simulink model "Ev3Model"  (R2019a)
settings: Solver=VariableStepAuto  StartTime=0.0  StopTime=40  RelTol=1e-3
values from neighbouring files (symbols this model uses):
  A = [0 1 0 0 ... (first row only)    [BEST.m]    (also in EV3Plant.m)
  Ac = A-B*K    [BEST.m]    (also in EV3Plant.m)
  B = [0;-m*l/d;0;(I+m*l^2)/d]    [BEST.m]    (also in EV3Plant.m)
  C = [1 0 0 0 ... (first row only)    [BEST.m]    (also in EV3Plant.m)
  D = [0 ... (first row only)    [BEST.m]    (also in EV3Plant.m)
  K = -[23.0811,2.5151,0.3162,1.0021]    [BEST.m]    (also in EV3Plant.m = lqr(A,B,Q,R))
  Kd = 0.005    [BEST.m]    (also in EV3Plant.m)
  Ki = 0.5    [BEST.m]    (also in EV3Plant.m)
  Kp = 1.5    [BEST.m]    (also in EV3Plant.m)
libraries: simulink x3
settings Model: Creator=mikiz  LastModifiedBy=mikiz
settings SolverCC: MaxConsecutiveMinStep=3  AlgebraicLoopSolver=LineSearch
settings DataIOCC: ReturnWorkspaceOutputs=off
settings DebuggingCC: ArithmeticOperatorsInVariantConditions=warning

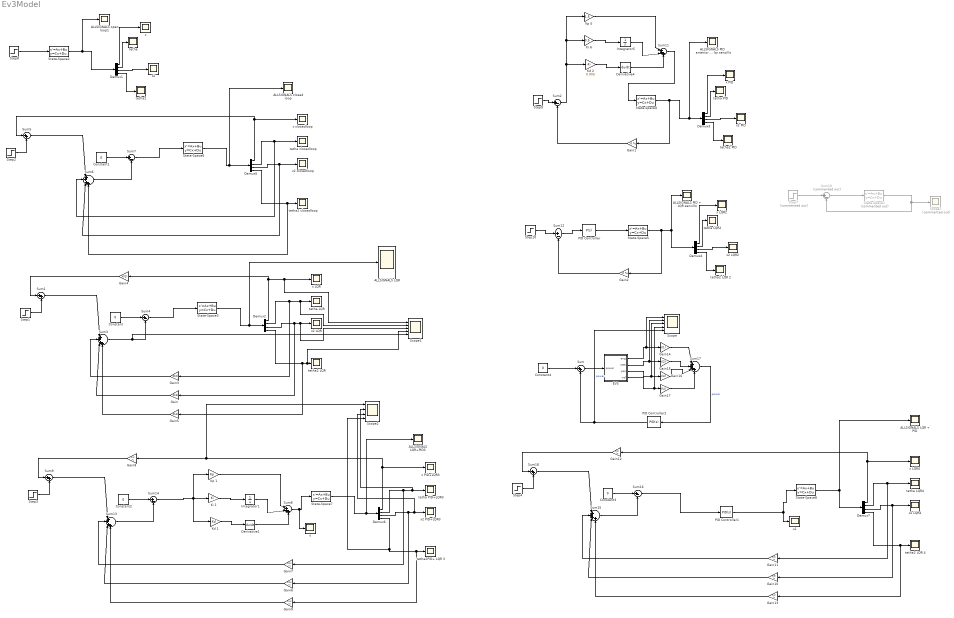
== system Ev3Model ==
  ALLSIGNALS LQR + PID : Scope
  "ALLSIGNALS PID + LQR sencillo " : Scope
  ALLSIGNALS PID anterior + lqr sencillo : Scope
  "ALLSIGNALS LQR " : Scope
  "ALLSIGNALS LQR+PIDS " : Scope
  ALLSIGNALS closed loop : Scope
  ALLSIGNALS open loop1 : Scope
  Constant{,1..4} (5 alike) : Constant  Value=0
  Demux{1..7} (7 alike) : Demux
  Derivative1 : Derivative
  Derivative4 : Derivative
  "EV3 " : Subsystem
  Gain : Gain  Gain=K(3)
  Gain1 : Gain  Gain=K  Multiplication=Matrix(K*u)
  Gain10 : Gain  Gain=K(3)  Multiplication=Matrix(K*u)
  Gain11 : Gain  Gain=K(2)  Multiplication=Matrix(K*u)
  Gain12 : Gain  Gain=K(1)  Multiplication=Matrix(K*u)
  Gain13 : Gain  Gain=K(4)  Multiplication=Matrix(K*u)
  Gain14 : Gain  Gain=K(1)
  Gain15 : Gain  Gain=K(2)
  Gain16 : Gain  Gain=K(3)
  Gain17 : Gain  Gain=K(4)
  Gain2 : Gain  Gain=K  Multiplication=Matrix(K*u)
  Gain3 : Gain  Gain=K(2)
  Gain4 : Gain  Gain=K(1)
  Gain5 : Gain  Gain=K(4)
  Gain6 : Gain  Gain=K(3)  Multiplication=Matrix(K*u)
  Gain7 : Gain  Gain=K(2)  Multiplication=Matrix(K*u)
  Gain8 : Gain  Gain=K(1)  Multiplication=Matrix(K*u)
  Gain9 : Gain  Gain=K(4)  Multiplication=Matrix(K*u)
  Integrator1 : Integrator
  Integrator5 : Integrator
  Kd 1 : Gain  Gain=Kd
  Kd 2 : Gain  Gain=0.005
  Ki 1 : Gain  Gain=Ki
  Ki 6 : Gain  Gain=0.5
  Kp 1 : Gain  Gain=Kp
  Kp 5 : Gain  Gain=1.5
  PID Controller : simulink/Continuous/PID Controller  Controller=P  Form=Parallel  TimeDomain=Continuous-time  SampleTime=-1  IntegratorMethod=Forward Euler  FilterMethod=Forward Euler  ControllerParametersSource=internal  P=25  I=0  D=0  UseFilter=on  N=100  TunerSelectOption=Transfer Function Based (PID Tuner App)  InitialConditionSource=internal  InitialConditionForIntegrator=0  InitialConditionForFilter=0  DifferentiatorICPrevScaledInput=0  ExternalReset=none  TrackingMode=off  Kt=1  LimitOutput=off  UpperSaturationLimit=inf  LowerSaturationLimit=-inf  LinearizeAsGain=on  AntiWindupMode=none  Kb=1  POutMin=[]  POutMax=[]  IOutMin=[]  IOutMax=[]  DOutMin=[]  DOutMax=[]  NOutMin=[]  NOutMax=[]  SumOutMin=[]  SumOutMax=[]  SaturationOutMin=[]  SaturationOutMax=[]  PParamMin=[]  PParamMax=[]  IParamMin=[]  IParamMax=[]  DParamMin=[]  DParamMax=[]  NParamMin=[]  NParamMax=[]  KbParamMin=[]  KbParamMax=[]  KtParamMin=[]  KtParamMax=[]  KbOutMin=[]  KbOutMax=[]  KtOutMin=[]  KtOutMax=[]  IntegratorOutMin=[]  IntegratorOutMax=[]  FilterOutMin=[]  FilterOutMax=[]  SumI1OutMin=[]  SumI1OutMax=[]  SumI2OutMin=[]  SumI2OutMax=[]  SumI3OutMin=[]  SumI3OutMax=[]  SumI4OutMin=[]  SumI4OutMax=[]  SumDOutMin=[]  SumDOutMax=[]  DifferentiatorOutMin=[]  DifferentiatorOutMax=[]  FilterDiffOutCoefMin=[]  FilterDiffOutCoefMax=[]  ReciprocalOutMin=[]  ReciprocalOutMax=[]  SumDenOutMin=[]  SumDenOutMax=[]  SumNumOutMin=[]  SumNumOutMax=[]  DivideOutMin=[]  DivideOutMax=[]  IntegratorContinuousStateAttributes=''  IntegratorStateMustResolveToSignalObject=off  IntegratorRTWStateStorageClass=Auto  FilterContinuousStateAttributes=''  FilterStateMustResolveToSignalObject=off  FilterRTWStateStorageClass=Auto  ParallelPVariant=InternalParameters  IdealPVariant=Disabled  IVariant=Disabled  DVariant=Disabled  IntegratorVariant=Disabled  SatVariant=Disabled  AWVariant=Disabled  PCopyVariant=Disabled  TRVariant=Disabled  FdbkBlocksVariant=Forward  IdealPFdbkVariant=Disabled  SatFdbkVariant=Disabled  DerivativeFilterVariant=Disabled  NVariant=Disabled  NCopyVariant=Disabled_SignalSpec  FilterICVariant=Disabled  IntegratorICVariant=Disabled  ExternalResetVariant=Disabled  TRSumVariant=Passthrough  SumFdbkVariant=Disabled  SumVariant=Passthrough_P
  PID Controller1 : simulink/Continuous/PID Controller  Controller=PID  Form=Parallel  TimeDomain=Continuous-time  SampleTime=-1  IntegratorMethod=Forward Euler  FilterMethod=Forward Euler  ControllerParametersSource=internal  P=3.727  I=24.1  D=-0.01253  UseFilter=on  N=66.27  TunerSelectOption=Transfer Function Based (PID Tuner App)  InitialConditionSource=internal  InitialConditionForIntegrator=0  InitialConditionForFilter=0  DifferentiatorICPrevScaledInput=0  ExternalReset=none  TrackingMode=off  Kt=1  LimitOutput=off  UpperSaturationLimit=inf  LowerSaturationLimit=-inf  LinearizeAsGain=on  AntiWindupMode=none  Kb=1  POutMin=[]  POutMax=[]  IOutMin=[]  IOutMax=[]  DOutMin=[]  DOutMax=[]  NOutMin=[]  NOutMax=[]  SumOutMin=[]  SumOutMax=[]  SaturationOutMin=[]  SaturationOutMax=[]  PParamMin=[]  PParamMax=[]  IParamMin=[]  IParamMax=[]  DParamMin=[]  DParamMax=[]  NParamMin=[]  NParamMax=[]  KbParamMin=[]  KbParamMax=[]  KtParamMin=[]  KtParamMax=[]  KbOutMin=[]  KbOutMax=[]  KtOutMin=[]  KtOutMax=[]  IntegratorOutMin=[]  IntegratorOutMax=[]  FilterOutMin=[]  FilterOutMax=[]  SumI1OutMin=[]  SumI1OutMax=[]  SumI2OutMin=[]  SumI2OutMax=[]  SumI3OutMin=[]  SumI3OutMax=[]  SumI4OutMin=[]  SumI4OutMax=[]  SumDOutMin=[]  SumDOutMax=[]  DifferentiatorOutMin=[]  DifferentiatorOutMax=[]  FilterDiffOutCoefMin=[]  FilterDiffOutCoefMax=[]  ReciprocalOutMin=[]  ReciprocalOutMax=[]  SumDenOutMin=[]  SumDenOutMax=[]  SumNumOutMin=[]  SumNumOutMax=[]  DivideOutMin=[]  DivideOutMax=[]  IntegratorContinuousStateAttributes=''  IntegratorStateMustResolveToSignalObject=off  IntegratorRTWStateStorageClass=Auto  FilterContinuousStateAttributes=''  FilterStateMustResolveToSignalObject=off  FilterRTWStateStorageClass=Auto  ParallelPVariant=InternalParameters  IdealPVariant=Disabled  IVariant=InternalParameters  DVariant=InternalParameters  IntegratorVariant=Continuous  SatVariant=Disabled  AWVariant=Passthrough  PCopyVariant=Disabled  TRVariant=Disabled  FdbkBlocksVariant=Forward  IdealPFdbkVariant=Disabled  SatFdbkVariant=Disabled  DerivativeFilterVariant=ContFilter  NVariant=InternalParameters  NCopyVariant=Disabled  FilterICVariant=InternalICsFilter  IntegratorICVariant=InternalICs  ExternalResetVariant=Disabled  TRSumVariant=Passthrough  SumFdbkVariant=Disabled  SumVariant=Sum_PID
  PID Controller2 : simulink/Continuous/PID Controller  Controller=PID  Form=Parallel  TimeDomain=Continuous-time  SampleTime=-1  IntegratorMethod=Forward Euler  FilterMethod=Forward Euler  ControllerParametersSource=internal  P=Kp  I=Ki  D=Kd  UseFilter=on  N=100  TunerSelectOption=Transfer Function Based (PID Tuner App)  InitialConditionSource=internal  InitialConditionForIntegrator=0  InitialConditionForFilter=0  DifferentiatorICPrevScaledInput=0  ExternalReset=none  TrackingMode=off  Kt=1  LimitOutput=off  UpperSaturationLimit=inf  LowerSaturationLimit=-inf  LinearizeAsGain=on  AntiWindupMode=none  Kb=1  POutMin=[]  POutMax=[]  IOutMin=[]  IOutMax=[]  DOutMin=[]  DOutMax=[]  NOutMin=[]  NOutMax=[]  SumOutMin=[]  SumOutMax=[]  SaturationOutMin=[]  SaturationOutMax=[]  PParamMin=[]  PParamMax=[]  IParamMin=[]  IParamMax=[]  DParamMin=[]  DParamMax=[]  NParamMin=[]  NParamMax=[]  KbParamMin=[]  KbParamMax=[]  KtParamMin=[]  KtParamMax=[]  KbOutMin=[]  KbOutMax=[]  KtOutMin=[]  KtOutMax=[]  IntegratorOutMin=[]  IntegratorOutMax=[]  FilterOutMin=[]  FilterOutMax=[]  SumI1OutMin=[]  SumI1OutMax=[]  SumI2OutMin=[]  SumI2OutMax=[]  SumI3OutMin=[]  SumI3OutMax=[]  SumI4OutMin=[]  SumI4OutMax=[]  SumDOutMin=[]  SumDOutMax=[]  DifferentiatorOutMin=[]  DifferentiatorOutMax=[]  FilterDiffOutCoefMin=[]  FilterDiffOutCoefMax=[]  ReciprocalOutMin=[]  ReciprocalOutMax=[]  SumDenOutMin=[]  SumDenOutMax=[]  SumNumOutMin=[]  SumNumOutMax=[]  DivideOutMin=[]  DivideOutMax=[]  IntegratorContinuousStateAttributes=''  IntegratorStateMustResolveToSignalObject=off  IntegratorRTWStateStorageClass=Auto  FilterContinuousStateAttributes=''  FilterStateMustResolveToSignalObject=off  FilterRTWStateStorageClass=Auto  ParallelPVariant=InternalParameters  IdealPVariant=Disabled  IVariant=InternalParameters  DVariant=InternalParameters  IntegratorVariant=Continuous  SatVariant=Disabled  AWVariant=Passthrough  PCopyVariant=Disabled  TRVariant=Disabled  FdbkBlocksVariant=Forward  IdealPFdbkVariant=Disabled  SatFdbkVariant=Disabled  DerivativeFilterVariant=ContFilter  NVariant=InternalParameters  NCopyVariant=Disabled  FilterICVariant=InternalICsFilter  IntegratorICVariant=InternalICs  ExternalResetVariant=Disabled  TRSumVariant=Passthrough  SumFdbkVariant=Disabled  SumVariant=Sum_PID
  Scope : Scope  NumInputPorts=5
  Scope1 : Scope  NumInputPorts=5
  Scope2 : Scope  NumInputPorts=4
  Scope7 : Scope  Commented=on
  State-Space1 : StateSpace  Commented=on  A=A  B=B  C=C  D=D  InitialCondition=0
  State-Space2 : StateSpace  A=A  B=B  C=C  D=D  InitialCondition=0
  State-Space{3..5,7..8} (5 alike) : StateSpace  A=Ac  B=B  C=C  D=D  InitialCondition=0
  State-Space6 : StateSpace  A=A  B=B  C=C  D=D  InitialCondition=0
  Step{1..4,8} (5 alike) : Step  SampleTime=0
  Step10 : Step  After=0.08  SampleTime=0
  Step7 : Step  Commented=on  SampleTime=0
  Step9 : Step  After=0.08  SampleTime=0
  Sum{,1,5,9,18} (5 alike) : Sum  Inputs=|++
  Sum10 : Sum  Commented=on  Inputs=|+-
  Sum11 : Sum  Inputs=|+++
  Sum{2,4,7,12,14,16} (6 alike) : Sum  Inputs=|+-
  Sum{3,6,13,15,17} (5 alike) : Sum  Inputs=|++++
  Sum8 : Sum  Inputs=|+++
  tetha : Scope
  tetha LQR : Scope
  tetha LQR2 : Scope
  tetha LQR4 : Scope
  tetha PID : Scope
  tetha PID+LQR3 : Scope
  tetha closedloop : Scope
  tetha2 : Scope
  "tetha2 LQR " : Scope
  tetha2 LQR 2 : Scope
  tetha2 LQR 4 : Scope
  tetha2 PID : Scope
  tetha2 closedloop : Scope
  tetha2PID+ LQR 3 : Scope
  u : Scope
  u1 : Scope
  x : Scope
  x LQR : Scope
  x LQR2 : Scope
  x LQR4 : Scope
  x PID : Scope
  x PID+LQR3 : Scope
  x closedloop : Scope
  x2 : Scope
  x2 LQR : Scope
  x2 LQR2 : Scope
  x2 LQR4 : Scope
  x2 PID : Scope
  x2 PID+LQR3 : Scope
  x2 closedloop : Scope
  wires:
  State-Space1/1 -> Scope7/1, Sum10/2
  Step7/1 -> Sum10/1
  Sum10/1 -> State-Space1/1
  Step8/1 -> State-Space2/1
  Demux1/4 -> tetha2/1
  Demux1/3 -> x2/1
  Demux1/2 -> tetha/1
  Demux1/1 -> x/1
  State-Space2/1 -> ALLSIGNALS open loop1/1, Demux1/1
  Demux2/4 -> Gain5/1, Scope1/4, "tetha2 LQR "/1
  Demux2/2 -> Gain3/1, Scope1/2, tetha LQR/1
  Demux2/3 -> Gain/1, Scope1/3, x2 LQR/1
  State-Space3/1 -> "ALLSIGNALS LQR "/1, Demux2/1
  Demux2/1 -> Gain4/1, Scope1/1, x LQR/1
  Step9/1 -> Sum2/1
  Demux3/1 -> x PID/1
  Demux3/4 -> tetha2 PID/1
  State-Space4/1 -> Gain1/1, ALLSIGNALS PID anterior + lqr sencillo/1, Demux3/1
  Demux3/3 -> x2 PID/1
  Demux3/2 -> tetha PID/1
  Gain1/1 -> Sum2/2
  Sum11/1 -> State-Space4/1
  Derivative4/1 -> Sum11/3
  Kp 5/1 -> Sum11/1
  Integrator5/1 -> Sum11/2
  Sum2/1 -> Ki 6/1, Kp 5/1, Kd 2/1
  Ki 6/1 -> Integrator5/1
  Kd 2/1 -> Derivative4/1
  Step10/1 -> Sum12/1
  Demux4/1 -> x LQR2/1
  Demux4/4 -> tetha2 LQR 2/1
  State-Space5/1 -> Gain2/1, Demux4/1, "ALLSIGNALS PID + LQR sencillo "/1
  Demux4/3 -> x2 LQR2/1
  Demux4/2 -> tetha LQR2/1
  Gain2/1 -> Sum12/2
  Sum12/1 -> PID Controller/1
  PID Controller/1 -> State-Space5/1
  Sum1/1 -> Sum3/1
  Gain4/1 -> Sum1/1
  Step1/1 -> Sum1/2
  Constant/1 -> Sum4/1
  Gain3/1 -> Sum3/2
  Gain/1 -> Sum3/3
  Gain5/1 -> Sum3/4
  Sum3/1 -> Scope1/5, Sum4/2
  Sum4/1 -> State-Space3/1
  Demux5/4 -> Sum6/4, tetha2 closedloop/1
  Demux5/3 -> Sum6/3, x2 closedloop/1
  Sum6/1 -> Sum7/2
  Constant1/1 -> Sum7/1
  Demux5/1 -> Sum5/1, x closedloop/1
  Demux5/2 -> Sum6/2, tetha closedloop/1
  Sum7/1 -> State-Space6/1
  State-Space6/1 -> ALLSIGNALS closed loop/1, Demux5/1
  Sum5/1 -> Sum6/1
  Step2/1 -> Sum5/2
  Kp 1/1 -> Sum8/1
  Ki 1/1 -> Integrator1/1
  Integrator1/1 -> Sum8/2
  Derivative1/1 -> Sum8/3
  Gain7/1 -> Sum13/2
  Kd 1/1 -> Derivative1/1
  Gain9/1 -> Sum13/4
  Gain6/1 -> Sum13/3
  Sum13/1 -> Sum14/2
  Constant2/1 -> Sum14/1
  Gain8/1 -> Sum9/1
  Demux6/1 -> Scope2/1, Gain8/1, x PID+LQR3/1
  Demux6/3 -> Gain6/1, Scope2/3, x2 PID+LQR3/1
  Demux6/2 -> Scope2/2, tetha PID+LQR3/1, Gain7/1
  State-Space7/1 -> "ALLSIGNALS LQR+PIDS "/1, Demux6/1
  Sum9/1 -> Sum13/1
  Demux6/4 -> tetha2PID+ LQR 3/1, Gain9/1, Scope2/4
  Step3/1 -> Sum9/2
  Sum14/1 -> Kd 1/1, Kp 1/1, Ki 1/1
  Sum8/1 -> u/1, State-Space7/1
  Gain12/1 -> Sum18/1
  Demux7/3 -> Gain10/1, x2 LQR4/1
  Step4/1 -> Sum18/2
  Sum18/1 -> Sum15/1
  Gain11/1 -> Sum15/2
  Demux7/2 -> Gain11/1, tetha LQR4/1
  State-Space8/1 -> Demux7/1, ALLSIGNALS LQR + PID/1
  Constant3/1 -> Sum16/1
  PID Controller1/1 -> State-Space8/1, u1/1
  Demux7/1 -> Gain12/1, x LQR4/1
  Demux7/4 -> Gain13/1, tetha2 LQR 4/1
  Gain13/1 -> Sum15/4
  Sum15/1 -> Sum16/2
  Gain10/1 -> Sum15/3
  Sum16/1 -> PID Controller1/1
  PID Controller2/1 -> Scope/5, Sum/2  "power"
  Gain16/1 -> Sum17/3
  "EV3 "/4(vel) -> Scope/4, Gain17/1
  "EV3 "/3(pos) -> Gain16/1, Scope/3
  "EV3 "/1(ang) -> Scope/1, Gain14/1
  Gain15/1 -> Sum17/2
  Gain17/1 -> Sum17/4
  "EV3 "/2(rate) -> Gain15/1, Scope/2
  Gain14/1 -> Sum17/1
  Sum/1 -> "EV3 "/1(power)
  Sum17/1 -> PID Controller2/1  "power"
  Constant4/1 -> Sum/1

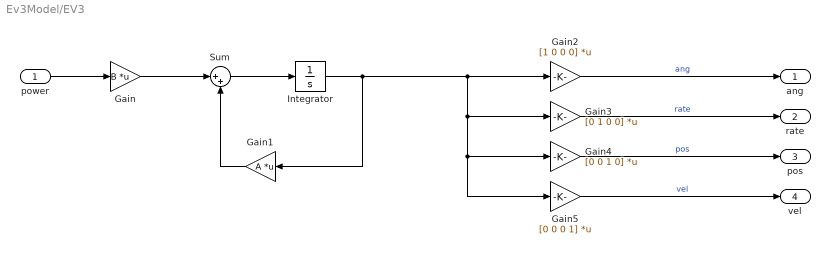
== system Ev3Model/EV3  ==
  power : Inport
  Gain : Gain  Gain=B  Multiplication=Matrix(K*u)
  Gain1 : Gain  Gain=A  Multiplication=Matrix(K*u)
  Gain2 : Gain  Gain=[1 0 0 0]  Multiplication=Matrix(K*u)
  Gain3 : Gain  Gain=[0 1 0 0]  Multiplication=Matrix(K*u)
  Gain4 : Gain  Gain=[0 0 1 0]  Multiplication=Matrix(K*u)
  Gain5 : Gain  Gain=[0 0 0 1]  Multiplication=Matrix(K*u)
  Integrator : Integrator
  Sum : Sum  Inputs=|++
  ang : Outport
  rate : Outport  Port=2
  pos : Outport  Port=3
  vel : Outport  Port=4
  wires:
  Gain1/1 -> Sum/2
  Gain/1 -> Sum/1
  Sum/1 -> Integrator/1
  Integrator/1 -> Gain1/1, Gain2/1, Gain3/1, Gain4/1, Gain5/1
  power/1 -> Gain/1
  Gain4/1 -> pos/1  "pos"
  Gain3/1 -> rate/1  "rate"
  Gain5/1 -> vel/1  "vel"
  Gain2/1 -> ang/1  "ang"
